simulink model "Signal_Adder_SimulinkFile"  (R2020a)
settings: Solver=VariableStepAuto  StartTime=0.0  StopTime=10.0  MaxStep=0.01  RelTol=1e-3
settings Model: Creator=alexd  LastModifiedBy=alexd

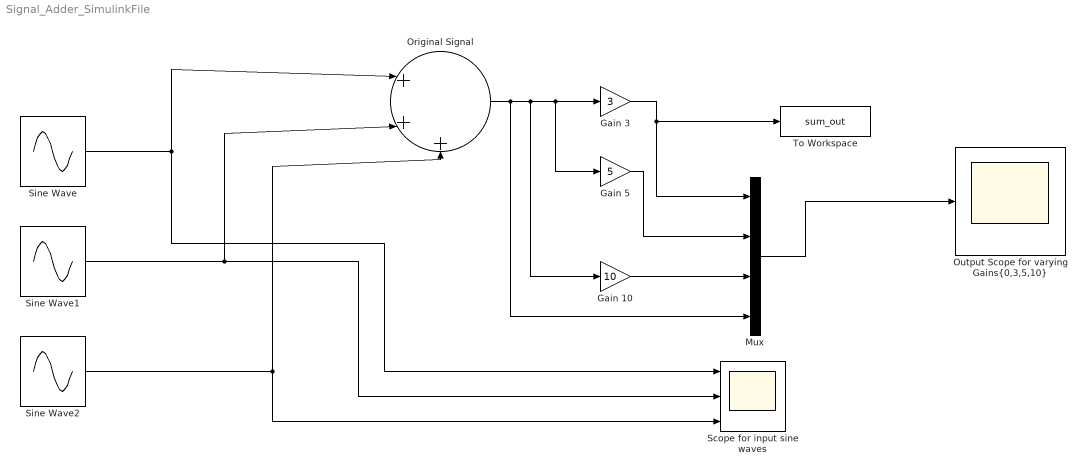
== system Signal_Adder_SimulinkFile ==
  Gain 10 : Gain  Gain=10
  Gain 3 : Gain  Gain=3
  Gain 5 : Gain  Gain=5
  Mux : Mux
  Original Signal : Sum  Inputs=|+++
  "Output Scope for varying Gains{0,3,5,10}" : Scope
  Scope for input sine waves : Scope  NumInputPorts=3
  Sine Wave : Sin  SampleTime=0
  Sine Wave1 : Sin  Frequency=5  SampleTime=0
  Sine Wave2 : Sin  Frequency=10  SampleTime=0
  To Workspace : ToWorkspace  VariableName=sum_out  SaveFormat=Timeseries  SampleTime=-1
  wires:
  Sine Wave/1 -> Scope for input sine waves/1, Original Signal/1
  Sine Wave2/1 -> Scope for input sine waves/3, Original Signal/3
  Sine Wave1/1 -> Scope for input sine waves/2, Original Signal/2
  Original Signal/1 -> Mux/4, Gain 10/1, Gain 5/1, Gain 3/1
  Gain 3/1 -> Mux/1, To Workspace/1
  Mux/1 -> "Output Scope for varying Gains{0,3,5,10}"/1
  Gain 5/1 -> Mux/2
  Gain 10/1 -> Mux/3
